simulink model "Zad_5_sch"  (R2022a)
settings: Solver=VariableStepAuto  StartTime=0.0  StopTime=10.0  RelTol=1e-3
model workspace (MAT data in the model file):
  A = [0  1  0; 3198.8547998  0  -49.6726703592; 0  0  -186.260159523]
  B = [0  0; 0  9.81; 468.723691441  0]
  C = [1 0 0]
  D = [0 0]
  L = [113.739840477 12013.6539685 12921.50985]
  Tp = 0.01
values from neighbouring files (symbols this model uses):
  a21 = (1/(2*m))*x30^2*(FemP1/FemP2^2)*exp(-x10/FemP2)    [Zad_2.m]
  a23 = -(1/m)*x30*(FemP1/FemP2)*exp(-x10/FemP2)    [Zad_2.m]
  a31 = (1/f1)*exp(x10/f2)*(ki*u10+ci-x30)    [Zad_2.m]
  a33 = -(f2/f1)*exp(x10/f2)    [Zad_2.m]
  b31 = ki*(f2/f1)*exp(x10/f2)    [Zad_2.m]
  g = 9.81    [Zad_2.m]
  K1 = 1    [Zad_4.m]
  K3g = -1/a23    [Zad_4.m]
  K3yr = -a21/a23    [Zad_4.m]
  Kg = a33/(a23*b31)    [Zad_4.m]
  Kxpom = place(A,Bpom,p_d)    [Zad_4.m]    (also in Zad_5.m; Zad_6.m)
  Kyr = (a21*a33-a31*a23)/(a23*b31)    [Zad_4.m]
  xd = d-bd    (= 0.01326)    [Zad_2.m]
settings Model: Creator=marci  LastModifiedBy=marci

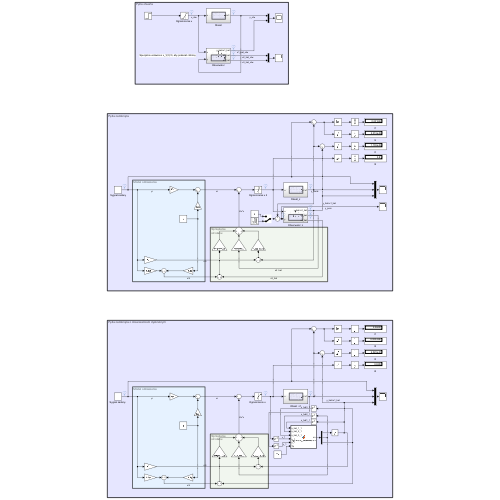
[thumbnail: Simulink's stored preview of the top-level diagram]
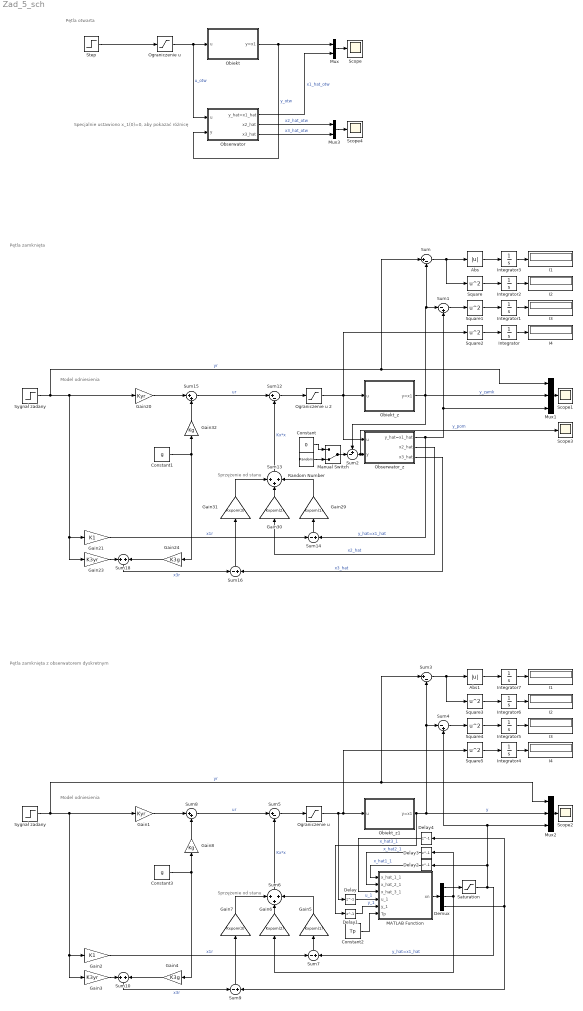
== system Zad_5_sch ==
  note: Specjalnie ustawiono x_1(0)=0, aby pokazać różnicę
  note: Pętla zamknięta
  note: Pętla otwarta
  note: Model odniesienia
  note: Sprzężenie
      | od stanu
  note: Pętla zamknięta z obserwatorem dyskretnym
  note: Model odniesienia
  note: Sprzężenie
      | od stanu
  " Sygnał zadany" : Step  Time=0  After=0.008  SampleTime=0
  " Sygnał zadany  " : Step  Time=0  After=0.008  SampleTime=0
  Abs : Abs  SaturateOnIntegerOverflow=off
  Abs1 : Abs  SaturateOnIntegerOverflow=off
  Constant : Constant  Value=0
  Constant1 : Constant  Value=g
  Constant2 : Constant  Value=Tp
  Constant3 : Constant  Value=g
  Delay{,1,3..4} (4 alike) : Delay  DelayLength=1
  Delay2 : Delay  DelayLength=1  InitialCondition=xd
  Demux : Demux  Outputs=3
  Gain1 : Gain  Gain=Kyr
  Gain2 : Gain  Gain=K1
  Gain20 : Gain  Gain=Kyr
  Gain21 : Gain  Gain=K1
  Gain23 : Gain  Gain=K3yr
  Gain24 : Gain  Gain=K3g
  Gain29 : Gain  Gain=Kxpom(1)
  Gain3 : Gain  Gain=K3yr
  Gain30 : Gain  Gain=Kxpom(2)
  Gain31 : Gain  Gain=Kxpom(3)
  Gain32 : Gain  Gain=Kg
  Gain4 : Gain  Gain=K3g
  Gain5 : Gain  Gain=Kxpom(1)
  Gain6 : Gain  Gain=Kxpom(2)
  Gain7 : Gain  Gain=Kxpom(3)
  Gain8 : Gain  Gain=Kg
  I{1..4} (4 alike) : Display
  "I1 " : Display
  "I2 " : Display
  "I3 " : Display
  "I4 " : Display
  Integrator{,1..7} (8 alike) : Integrator
  MATLAB Function : MATLAB Function  TreatAsAtomicUnit=on
  Manual Switch : ManualSwitch  CurrentSetting=0
  Mux : Mux  Inputs=2
  Mux1 : Mux  Inputs=3
  Mux2 : Mux  Inputs=3
  Mux3 : Mux  Inputs=2
  Obiekt : Subsystem
  Obiekt_z : Subsystem
  Obiekt_z1 : Subsystem
  Obserwator : Subsystem
  Obserwator_z : Subsystem
  "Ograniczenie u " : Saturate  UpperLimit=1  LowerLimit=0  ZeroCross=off
  "Ograniczenie u  " : Saturate  UpperLimit=1  LowerLimit=0  ZeroCross=off
  Ograniczenie u 2 : Saturate  UpperLimit=1  LowerLimit=0  ZeroCross=off
  Random Number : RandomNumber  Variance=0.0000001  SampleTime=0.0001
  Saturation : Saturate  UpperLimit=xd  LowerLimit=0
  Scope{,1..4} (5 alike) : Scope
  Square{,1..5} (6 alike) : Math  Operator=square
  Step : Step  Time=0  SampleTime=0
  Sum{,3,5,12} (4 alike) : Sum  Inputs=|+-
  Sum1 : Sum  Inputs=|-+
  Sum10 : Sum
  Sum13 : Sum  Inputs=+++
  Sum{7,9,14,16} (4 alike) : Sum  Inputs=-+
  Sum15 : Sum  Inputs=|++
  Sum18 : Sum
  Sum2 : Sum  Inputs=+-|
  Sum4 : Sum  Inputs=|-+
  Sum6 : Sum  Inputs=+++
  Sum8 : Sum  Inputs=|++
  wires:
  "Ograniczenie u "/1 -> Obserwator/1(u), Obiekt/1(u)  "u_otw"
  Obiekt/1(y=x1) -> Obserwator/2(y), Mux/1  "y_otw"
  Step/1 -> "Ograniczenie u "/1
  Obserwator/1(y_hat=x1_hat) -> Mux/2  "x1_hat_otw"
  " Sygnał zadany"/1 -> Sum/1, Mux1/1, Gain20/1, Gain23/1, Gain21/1  "yr"
  Gain32/1 -> Sum15/2
  Gain29/1 -> Sum13/3
  Gain30/1 -> Sum13/2
  Gain21/1 -> Sum14/1  "x1r"
  Sum14/1 -> Gain29/1
  Sum15/1 -> Sum12/1  "ur"
  Gain24/1 -> Sum18/2
  Mux1/1 -> Scope1/1
  Sum16/1 -> Gain31/1
  Constant1/1 -> Gain24/1, Gain32/1
  Gain20/1 -> Sum15/1
  Gain23/1 -> Sum18/1
  Gain31/1 -> Sum13/1
  Sum13/1 -> Sum12/2  "Kx*x"
  Sum18/1 -> Sum16/1  "x3r"
  Sum12/1 -> Ograniczenie u 2/1
  Ograniczenie u 2/1 -> Square2/1, Obserwator_z/1(u), Obiekt_z/1(u)
  Obiekt_z/1(y=x1) -> Mux1/2, Sum1/1, Sum/2, Sum2/1  "y_zamk"
  Obserwator_z/1(y_hat=x1_hat) -> Sum1/2, Mux1/3, Sum14/2  "y_hat=x1_hat"
  Obserwator_z/2(x2_hat) -> Gain30/1  "x2_hat"
  Obserwator_z/3(x3_hat) -> Sum16/2  "x3_hat"
  Integrator/1 -> I4/1
  Integrator1/1 -> I3/1
  Integrator2/1 -> I2/1
  Integrator3/1 -> I1/1
  Abs/1 -> Integrator3/1
  Square/1 -> Integrator2/1
  Square2/1 -> Integrator/1
  Square1/1 -> Integrator1/1
  Sum/1 -> Square/1, Abs/1
  Sum1/1 -> Square1/1
  Sum2/1 -> Scope3/1, Obserwator_z/2(y)  "y_pom"
  Random Number/1 -> Manual Switch/2
  Manual Switch/1 -> Sum2/2
  Constant/1 -> Manual Switch/1
  Integrator4/1 -> "I4 "/1
  Obiekt_z1/1(y=x1) -> Delay1/1, Sum4/1, Sum3/2, Mux2/2  "y"
  Gain2/1 -> Sum7/1  "x1r"
  Integrator6/1 -> "I2 "/1
  Abs1/1 -> Integrator7/1
  Gain3/1 -> Sum10/1
  Square3/1 -> Integrator6/1
  Gain7/1 -> Sum6/1
  Square5/1 -> Integrator4/1
  Constant3/1 -> Gain4/1, Gain8/1
  Saturation/1 -> Mux2/3, Sum4/2, Delay2/1, Sum7/2  "y_hat=x1_hat"
  "Ograniczenie u  "/1 -> Square5/1, Obiekt_z1/1(u), Delay/1
  Integrator5/1 -> "I3 "/1
  Sum8/1 -> Sum5/1  "ur"
  Gain1/1 -> Sum8/1
  Sum7/1 -> Gain5/1
  Gain4/1 -> Sum10/2
  " Sygnał zadany  "/1 -> Sum3/1, Mux2/1, Gain1/1, Gain3/1, Gain2/1  "yr"
  Sum4/1 -> Square4/1
  Sum10/1 -> Sum9/1  "x3r"
  Gain6/1 -> Sum6/2
  Sum6/1 -> Sum5/2  "Kx*x"
  Sum5/1 -> "Ograniczenie u  "/1
  Gain5/1 -> Sum6/3
  Square4/1 -> Integrator5/1
  Sum3/1 -> Square3/1, Abs1/1
  Gain8/1 -> Sum8/2
  Integrator7/1 -> "I1 "/1
  Mux2/1 -> Scope2/1
  Sum9/1 -> Gain7/1
  Delay1/1 -> MATLAB Function/5(y_1)  "y_1"
  Delay/1 -> MATLAB Function/4(u_1)  "u_1"
  Delay2/1 -> MATLAB Function/1(x_hat_1_1)  "x_hat1_1"
  Delay3/1 -> MATLAB Function/2(x_hat_2_1)  "x_hat2_1"
  Delay4/1 -> MATLAB Function/3(x_hat_3_1)  "x_hat3_1"
  MATLAB Function/1(xn) -> Demux/1
  Demux/2 -> Gain6/1, Delay3/1
  Demux/3 -> Delay4/1, Sum9/2
  Demux/1 -> Saturation/1
  Constant2/1 -> MATLAB Function/6(Tp)
  Mux/1 -> Scope/1
  Obserwator/2(x2_hat) -> Mux3/1  "x2_hat_otw"
  Obserwator/3(x3_hat) -> Mux3/2  "x3_hat_otw"
  Mux3/1 -> Scope4/1

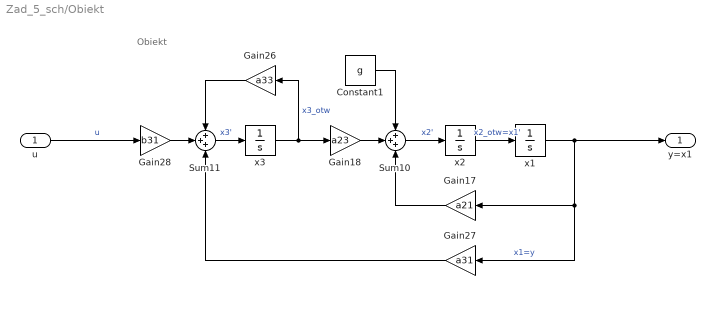
== system Zad_5_sch/Obiekt ==
  note: Obiekt
  u : Inport
  " x1" : Integrator  InitialCondition=xd  LimitOutput=on  UpperSaturationLimit=xd  LowerSaturationLimit=0
  " x2" : Integrator
  " x3" : Integrator
  Constant1 : Constant  Value=g
  Gain17 : Gain  Gain=a21
  Gain18 : Gain  Gain=a23
  Gain26 : Gain  Gain=a33
  Gain27 : Gain  Gain=a31
  Gain28 : Gain  Gain=b31
  Sum10 : Sum  Inputs=+++
  Sum11 : Sum  Inputs=+++
  y=x1 : Outport
  wires:
  Gain18/1 -> Sum10/2
  " x2"/1 -> " x1"/1  "x2_otw=x1'"
  u/1 -> Gain28/1  "u"
  " x1"/1 -> y=x1/1, Gain17/1, Gain27/1  "x1=y"
  Sum10/1 -> " x2"/1  "x2'"
  Gain28/1 -> Sum11/2
  Gain17/1 -> Sum10/3
  " x3"/1 -> Gain18/1, Gain26/1  "x3_otw"
  Constant1/1 -> Sum10/1
  Gain26/1 -> Sum11/1
  Gain27/1 -> Sum11/3
  Sum11/1 -> " x3"/1  "x3'"

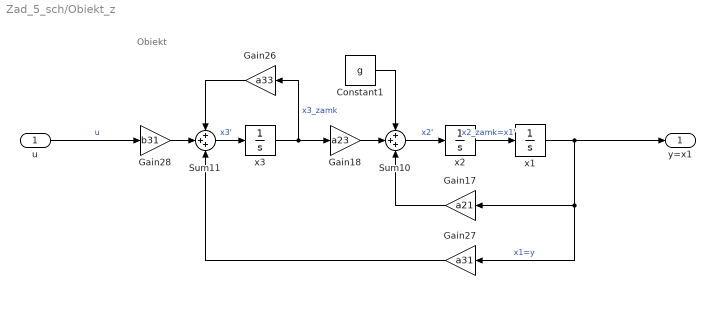
== system Zad_5_sch/Obiekt_z ==
  note: Obiekt
  u : Inport
  " x1" : Integrator  InitialCondition=xd  LimitOutput=on  UpperSaturationLimit=xd  LowerSaturationLimit=0
  " x2" : Integrator
  " x3" : Integrator
  Constant1 : Constant  Value=g
  Gain17 : Gain  Gain=a21
  Gain18 : Gain  Gain=a23
  Gain26 : Gain  Gain=a33
  Gain27 : Gain  Gain=a31
  Gain28 : Gain  Gain=b31
  Sum10 : Sum  Inputs=+++
  Sum11 : Sum  Inputs=+++
  y=x1 : Outport
  wires:
  Gain18/1 -> Sum10/2
  " x2"/1 -> " x1"/1  "x2_zamk=x1'"
  u/1 -> Gain28/1  "u"
  " x1"/1 -> y=x1/1, Gain17/1, Gain27/1  "x1=y"
  Sum10/1 -> " x2"/1  "x2'"
  Gain28/1 -> Sum11/2
  Gain17/1 -> Sum10/3
  " x3"/1 -> Gain18/1, Gain26/1  "x3_zamk"
  Constant1/1 -> Sum10/1
  Gain26/1 -> Sum11/1
  Gain27/1 -> Sum11/3
  Sum11/1 -> " x3"/1  "x3'"

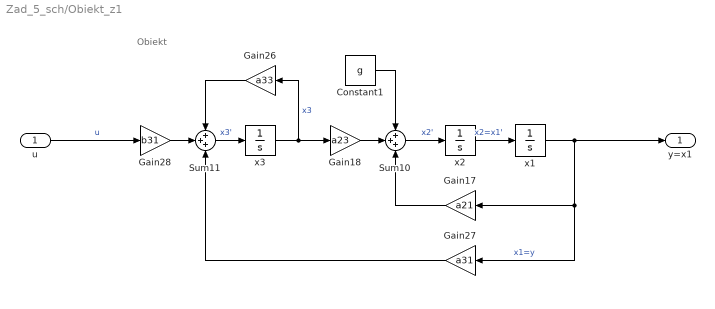
== system Zad_5_sch/Obiekt_z1 ==
  note: Obiekt
  u : Inport
  " x1" : Integrator  InitialCondition=xd  LimitOutput=on  UpperSaturationLimit=xd  LowerSaturationLimit=0
  " x2" : Integrator
  " x3" : Integrator
  Constant1 : Constant  Value=g
  Gain17 : Gain  Gain=a21
  Gain18 : Gain  Gain=a23
  Gain26 : Gain  Gain=a33
  Gain27 : Gain  Gain=a31
  Gain28 : Gain  Gain=b31
  Sum10 : Sum  Inputs=+++
  Sum11 : Sum  Inputs=+++
  y=x1 : Outport
  wires:
  Gain18/1 -> Sum10/2
  " x2"/1 -> " x1"/1  "x2=x1'"
  u/1 -> Gain28/1  "u"
  " x1"/1 -> y=x1/1, Gain17/1, Gain27/1  "x1=y"
  Sum10/1 -> " x2"/1  "x2'"
  Gain28/1 -> Sum11/2
  Gain17/1 -> Sum10/3
  " x3"/1 -> Gain18/1, Gain26/1  "x3"
  Constant1/1 -> Sum10/1
  Gain26/1 -> Sum11/1
  Gain27/1 -> Sum11/3
  Sum11/1 -> " x3"/1  "x3'"

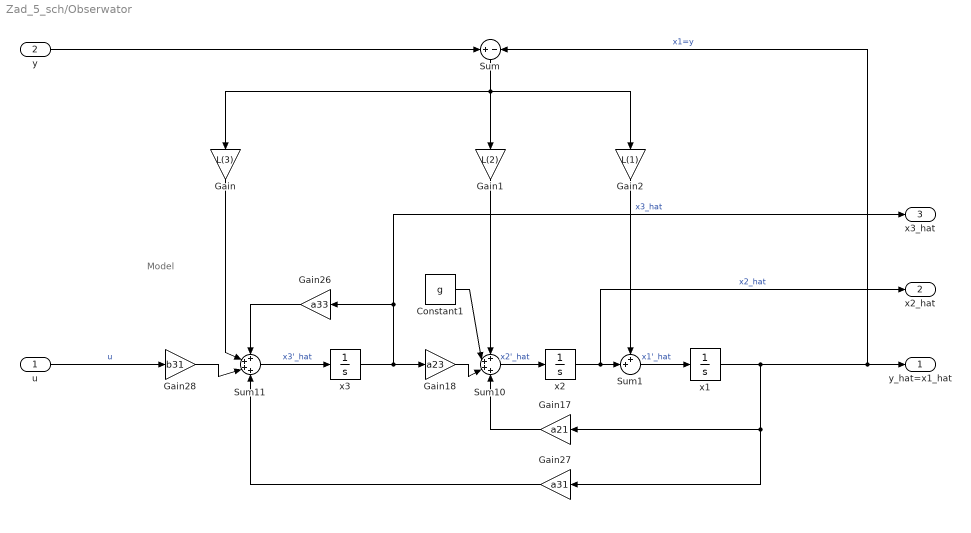
== system Zad_5_sch/Obserwator ==
  note: Model
  u : Inport
  y : Inport  Port=2
  " x1" : Integrator  LimitOutput=on  UpperSaturationLimit=xd  LowerSaturationLimit=0
  " x2" : Integrator
  " x3" : Integrator
  Constant1 : Constant  Value=g
  Gain : Gain  Gain=L(3)
  Gain1 : Gain  Gain=L(2)
  Gain17 : Gain  Gain=a21
  Gain18 : Gain  Gain=a23
  Gain2 : Gain  Gain=L(1)
  Gain26 : Gain  Gain=a33
  Gain27 : Gain  Gain=a31
  Gain28 : Gain  Gain=b31
  Sum : Sum  Inputs=+-
  Sum1 : Sum  Inputs=++|
  Sum10 : Sum  Inputs=++++
  Sum11 : Sum  Inputs=++++
  y_hat=x1_hat : Outport
  x2_hat : Outport  Port=2
  x3_hat : Outport  Port=3
  wires:
  Gain18/1 -> Sum10/3
  " x2"/1 -> x2_hat/1, Sum1/2  "x2_hat"
  u/1 -> Gain28/1  "u"
  " x1"/1 -> Sum/2, y_hat=x1_hat/1, Gain17/1, Gain27/1  "x1=y"
  Sum10/1 -> " x2"/1  "x2'_hat"
  Gain28/1 -> Sum11/3
  Gain17/1 -> Sum10/4
  " x3"/1 -> Gain18/1, Gain26/1, x3_hat/1  "x3_hat"
  Constant1/1 -> Sum10/2
  Gain26/1 -> Sum11/1
  Gain27/1 -> Sum11/4
  Sum11/1 -> " x3"/1  "x3'_hat"
  y/1 -> Sum/1
  Sum/1 -> Gain/1, Gain2/1, Gain1/1
  Gain/1 -> Sum11/2
  Gain1/1 -> Sum10/1
  Sum1/1 -> " x1"/1  "x1'_hat"
  Gain2/1 -> Sum1/1

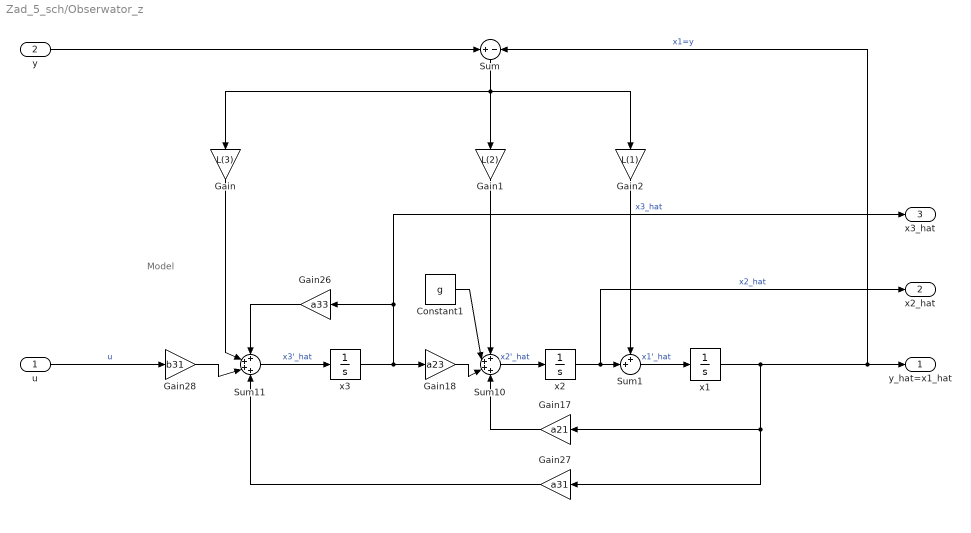
== system Zad_5_sch/Obserwator_z ==
  note: Model
  u : Inport
  y : Inport  Port=2
  " x1" : Integrator  InitialCondition=xd  LimitOutput=on  UpperSaturationLimit=xd  LowerSaturationLimit=0
  " x2" : Integrator
  " x3" : Integrator
  Constant1 : Constant  Value=g
  Gain : Gain  Gain=L(3)
  Gain1 : Gain  Gain=L(2)
  Gain17 : Gain  Gain=a21
  Gain18 : Gain  Gain=a23
  Gain2 : Gain  Gain=L(1)
  Gain26 : Gain  Gain=a33
  Gain27 : Gain  Gain=a31
  Gain28 : Gain  Gain=b31
  Sum : Sum  Inputs=+-
  Sum1 : Sum  Inputs=++|
  Sum10 : Sum  Inputs=++++
  Sum11 : Sum  Inputs=++++
  y_hat=x1_hat : Outport
  x2_hat : Outport  Port=2
  x3_hat : Outport  Port=3
  wires:
  Gain18/1 -> Sum10/3
  " x2"/1 -> x2_hat/1, Sum1/2  "x2_hat"
  u/1 -> Gain28/1  "u"
  " x1"/1 -> Sum/2, y_hat=x1_hat/1, Gain17/1, Gain27/1  "x1=y"
  Sum10/1 -> " x2"/1  "x2'_hat"
  Gain28/1 -> Sum11/3
  Gain17/1 -> Sum10/4
  " x3"/1 -> Gain18/1, Gain26/1, x3_hat/1  "x3_hat"
  Constant1/1 -> Sum10/2
  Gain26/1 -> Sum11/1
  Gain27/1 -> Sum11/4
  Sum11/1 -> " x3"/1  "x3'_hat"
  y/1 -> Sum/1
  Sum/1 -> Gain/1, Gain2/1, Gain1/1
  Gain/1 -> Sum11/2
  Gain1/1 -> Sum10/1
  Sum1/1 -> " x1"/1  "x1'_hat"
  Gain2/1 -> Sum1/1

== matlab function Zad_5_sch/MATLAB Function ==
  data: x_hat_1_1 input; xn output; x_hat_2_1 input; x_hat_3_1 input; u_1 input; y_1 input; Tp input
function xn=dyskretny_obserwator(x_hat_1_1, x_hat_2_1, x_hat_3_1, u_1, y_1,Tp)
%funkcja bedaca dyskretnym obserwatorem stanu
A=[0,1,0;3.198854799795517e+03,0,-49.672670359171390;0,0,-1.862601595234874e+02];
B=[0,0;0,9.810000000000000;4.687236914408560e+02,0];
C=[1,0,0];
L=[113.739840476513; 12013.6539684643; 12921.5098500384];

Tp1=Tp;

u_pom=[u_1; 1];
x_hat1=[x_hat_1_1; x_hat_2_1; x_hat_3_1];

%estymacja zmiennych stanu
xn = (eye(3)+A*Tp1)*x_hat1+B*Tp1*u_pom+L*Tp1*(y_1-C*x_hat1);
